simulink model "Hw1_2"  (R2015b)
settings: Solver=VariableStepAuto  StartTime=0.0  StopTime=500  RelTol=1e-3
settings Model: Creator=user  LastModifiedBy=user

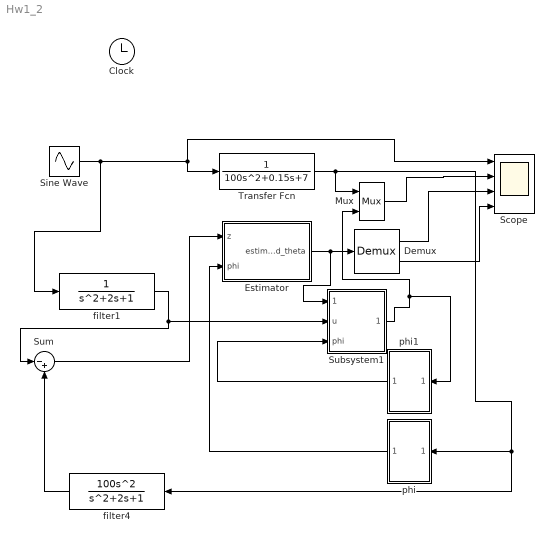
== system Hw1_2 ==
  Clock : Clock
      settings: Decimation=250
  Demux : Demux  Outputs=2
  Estimator : Subsystem
      mask Display: disp('Parameter\nEstimation')
  Mux : Mux  Inputs=2
  Scope : Scope  NumInputPorts=4
  Sine Wave : Sin  Bias=1  Frequency=pi/3  Phase=pi/2  SampleTime=0
  Subsystem1 : Subsystem
  Sum : Sum  Inputs=|-+
  Transfer Fcn : TransferFcn  Denominator=[100 0.15 7]
  filter1 : TransferFcn
  filter4 : TransferFcn  Numerator=[100 0 0]
  phi : Subsystem
  phi1 : Subsystem
  wires:
  Sine Wave/1 -> filter1/1, Transfer Fcn/1, Scope/1
  phi/1(Out1) -> Estimator/2(phi)
  Transfer Fcn/1 -> Mux/1, phi/1(In1), filter4/1
  filter4/1 -> Sum/2
  filter1/1 -> Sum/1, Subsystem1/2(u)
  Sum/1 -> Estimator/1(z)
  Estimator/1(estimated_theta) -> Subsystem1/1(theta_hat), Demux/1
  Demux/1 -> Scope/3
  Demux/2 -> Scope/4
  Mux/1 -> Scope/2
  Subsystem1/1(x_hat) -> phi1/1(In1), Mux/2
  phi1/1(Out1) -> Subsystem1/3(phi)

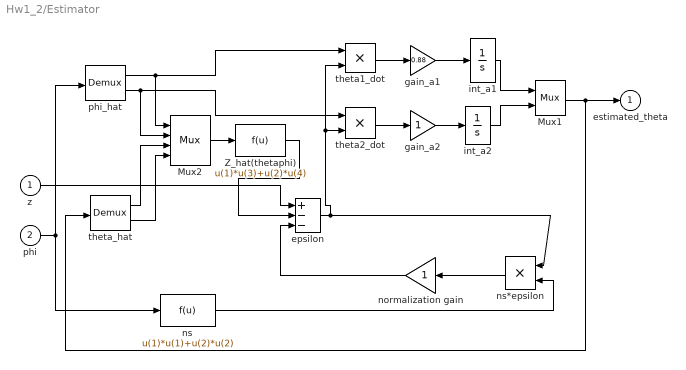
== system Hw1_2/Estimator ==
  z : Inport
  phi : Inport  Port=2
  Mux1 : Mux  Inputs=2
  Mux2 : Mux
  Z_hat(thetaphi) : Fcn  Expr=u(1)*u(3)+u(2)*u(4)
  epsilon : Sum  Inputs=+--  SaturateOnIntegerOverflow=on  InputSameDT=on  OutDataTypeStr=Inherit: Same as first input
  gain_a1 : Gain  Gain=0.88  SaturateOnIntegerOverflow=on  OutDataTypeStr=Inherit: Same as input  ParamDataTypeStr=Inherit: Same as input
  gain_a2 : Gain  SaturateOnIntegerOverflow=on  OutDataTypeStr=Inherit: Same as input  ParamDataTypeStr=Inherit: Same as input
  int_a1 : Integrator
  int_a2 : Integrator
  normalization gain : Gain  SaturateOnIntegerOverflow=on  OutDataTypeStr=Inherit: Same as input  ParamDataTypeStr=Inherit: Same as input
  ns : Fcn  Expr=u(1)*u(1)+u(2)*u(2)
      mask Display: disp('phi ''phi')
  ns*epsilon : Product  SaturateOnIntegerOverflow=on  RndMeth=Zero  InputSameDT=on  OutDataTypeStr=Inherit: Same as first input
  phi_hat : Demux  Outputs=2
  theta1_dot : Product  SaturateOnIntegerOverflow=on  RndMeth=Zero  InputSameDT=on  OutDataTypeStr=Inherit: Same as first input
  theta2_dot : Product  SaturateOnIntegerOverflow=on  RndMeth=Zero  InputSameDT=on  OutDataTypeStr=Inherit: Same as first input
  theta_hat : Demux  Outputs=2
  estimated_theta : Outport
  wires:
  z/1 -> epsilon/1
  normalization gain/1 -> epsilon/3
  phi_hat/1 -> theta1_dot/1, Mux2/1
  phi_hat/2 -> theta2_dot/1, Mux2/2
  Mux1/1 -> estimated_theta/1, theta_hat/1
  Z_hat(thetaphi)/1 -> epsilon/2
  phi/1 -> ns/1, phi_hat/1
  epsilon/1 -> ns*epsilon/1, theta1_dot/2, theta2_dot/2
  ns*epsilon/1 -> normalization gain/1
  int_a1/1 -> Mux1/1
  int_a2/1 -> Mux1/2
  theta_hat/1 -> Mux2/3
  theta_hat/2 -> Mux2/4
  Mux2/1 -> Z_hat(thetaphi)/1
  theta2_dot/1 -> gain_a2/1
  gain_a2/1 -> int_a2/1
  theta1_dot/1 -> gain_a1/1
  gain_a1/1 -> int_a1/1
  ns/1 -> ns*epsilon/2

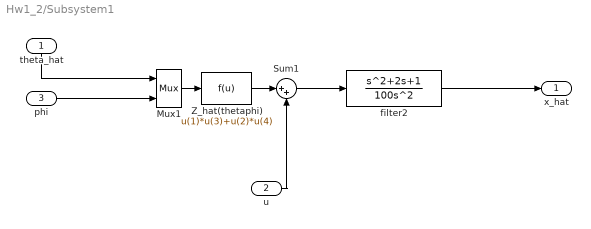
== system Hw1_2/Subsystem1 ==
  theta_hat : Inport
  u : Inport  Port=2
  phi : Inport  Port=3
  Mux1 : Mux  Inputs=2
  Sum1 : Sum  Inputs=|++
  Z_hat(thetaphi) : Fcn  Expr=u(1)*u(3)+u(2)*u(4)
  filter2 : TransferFcn  Numerator=[1 2 1]  Denominator=[100 0 0]
  x_hat : Outport
  wires:
  phi/1 -> Mux1/2
  u/1 -> Sum1/2
  theta_hat/1 -> Mux1/1
  filter2/1 -> x_hat/1
  Mux1/1 -> Z_hat(thetaphi)/1
  Sum1/1 -> filter2/1
  Z_hat(thetaphi)/1 -> Sum1/1

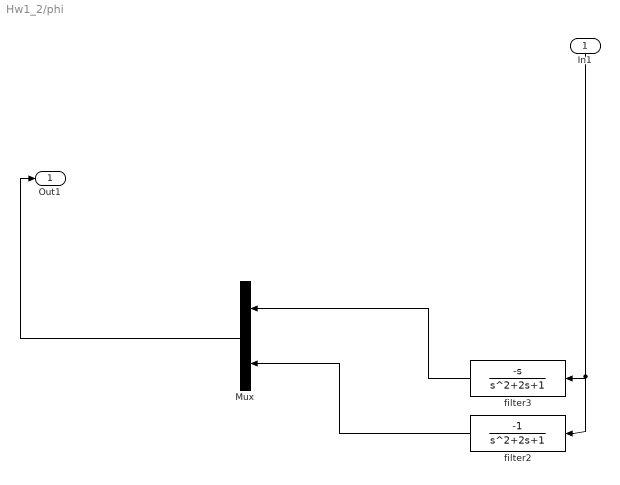
== system Hw1_2/phi ==
  In1 : Inport
  Mux : Mux  Inputs=2
  filter2 : TransferFcn  Numerator=[-1 ]
  filter3 : TransferFcn  Numerator="[-1  0]"
  Out1 : Outport
  wires:
  In1/1 -> filter2/1, filter3/1
  filter2/1 -> Mux/2
  Mux/1 -> Out1/1
  filter3/1 -> Mux/1

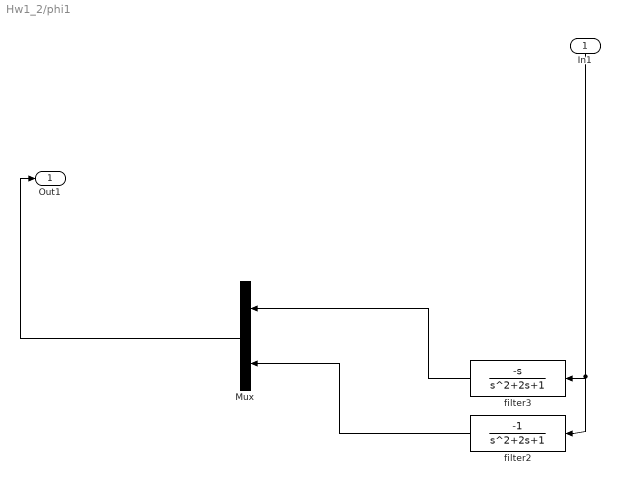
== system Hw1_2/phi1 ==
  In1 : Inport
  Mux : Mux  Inputs=2
  filter2 : TransferFcn  Numerator=[-1 ]
  filter3 : TransferFcn  Numerator="[-1  0]"
  Out1 : Outport
  wires:
  In1/1 -> filter2/1, filter3/1
  filter2/1 -> Mux/2
  Mux/1 -> Out1/1
  filter3/1 -> Mux/1
